simulink model "ev_ex_9"  (R2025a)
settings: Solver=VariableStepAuto  StartTime=0.0  StopTime=3600  RelTol=1e-3
undefined symbols (not defined in the file or in its folder): Ion, Lithium
libraries: spsBatteryLib x2, spsDiodeLib x2, spsIdealSwitchLib x2, spsSeriesRLCBranchLib x2, spsGroundLib x1, BatteryBalancing x1, sps_lib x1
settings Model: Creator=KRISHNA  LastModifiedBy=KRISHNA

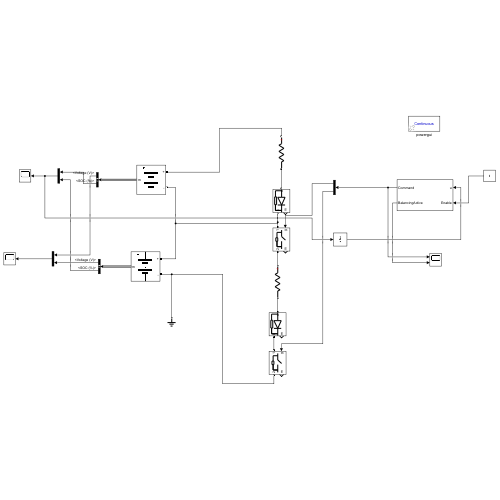
[thumbnail: Simulink's stored preview of the top-level diagram]
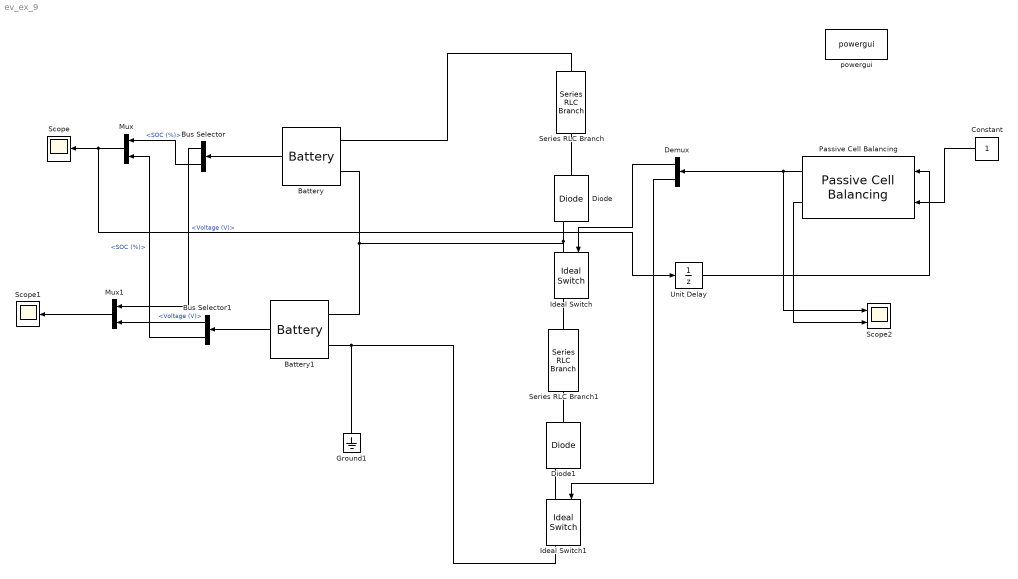
== system ev_ex_9 ==
  Battery : spsBatteryLib/Battery  BatType=Lithium-Ion  NomV=7.2  NomQ=5.4  SOC=90  Batt_Tr=1  PresetModel=on  MaxQ=5.4  MinV=5.4  FullV=8.3807  Dis_rate=2.3478  R=0.013333  Normal_OP=4.8835  expZone="[7.7788      0.2653]"
  Battery1 : spsBatteryLib/Battery  BatType=Lithium-Ion  NomV=7.2  NomQ=5.4  SOC=70  Batt_Tr=1  PresetModel=on  MaxQ=5.4  MinV=5.4  FullV=8.3807  Dis_rate=2.3478  R=0.013333  Normal_OP=4.8835  expZone="[7.7788      0.2653]"
  Bus Selector : BusSelector  OutputSignals=Voltage (V),SOC (%)
  Bus Selector1 : BusSelector  OutputSignals=Voltage (V),SOC (%)
  Constant : Constant
  Demux : Demux  Outputs=2
  Diode : spsDiodeLib/Diode  Ron=0.001  Lon=0  Vf=0.8  IC=0  UseSnubber=0  Rs=500  Cs=250e-9  Measurements=on
  Diode1 : spsDiodeLib/Diode  Ron=0.001  Lon=0  Vf=0.8  IC=0  UseSnubber=0  Rs=500  Cs=250e-9  Measurements=on
  Ground1 : spsGroundLib/Ground  LConnTagsString=a
  Ideal Switch : spsIdealSwitchLib/Ideal Switch  Ron=0.001  Lon=0  IC=0  Rs=1e5  Cs=inf  Measurements=on
  Ideal Switch1 : spsIdealSwitchLib/Ideal Switch  Ron=0.001  Lon=0  IC=0  Rs=1e5  Cs=inf  Measurements=on
  Mux : Mux  Inputs=2
  Mux1 : Mux  Inputs=2
  Passive Cell Balancing : BatteryBalancing/Passive Cell Balancing  Threshold=0.2  HysteresisBand=0  Td_on=1  Td_off=1  Ts=1  dataType=double
      settings: LibrarySourceBlock=batt_sl_lib/Cell Balancing/Passive Cell Balancing
  Scope : Scope
      settings: ActiveDisplayYMinimum=-10.40273292213508  ActiveDisplayYMaximum=101.52121489807514
  Scope1 : Scope
      settings: ActiveDisplayYMinimum=-0.97308129227086171  ActiveDisplayYMaximum=8.7577316304377568
  Scope2 : Scope  NumInputPorts=2
      settings: ActiveDisplayYMinimum=-0.12499999999999997  ActiveDisplayYMaximum=1.125  DataLoggingVariableName=ScopeData2
  Series RLC Branch : spsSeriesRLCBranchLib/Series RLC Branch  LConnTagsString=__new0  RConnTagsString=__new0  BranchType=R  Resistance=1  Inductance=1e-3  SetiL0=off  InitialCurrent=0  Capacitance=1e-6  Setx0=off  InitialVoltage=0  Measurements=None
  Series RLC Branch1 : spsSeriesRLCBranchLib/Series RLC Branch  LConnTagsString=__new0  RConnTagsString=__new0  BranchType=R  Resistance=1  Inductance=1e-3  SetiL0=off  InitialCurrent=0  Capacitance=1e-6  Setx0=off  InitialVoltage=0  Measurements=None
  Unit Delay : UnitDelay  SampleTime=-1  HasFrameUpgradeWarning=on
  powergui : sps_lib/powergui  Priority=1  SimulationMode=Continuous  SampleTime=50e-6  frequency=60  Iterations=50  frequencyindice=0  Pbase=100e6  ErrMax=1e-4  UnitsV=kV  UnitsW=MW  buscounter=0  FunctionMessages=off  echomessages=off  EnableUseOfTLC=off  CurrentSourceSwitches=off  DisableSnubberDevices=off  DisableRonSwitches=off  DisableVfSwitches=off  DisplayEquations=off  AutomaticDiscreteSolvers=off  SolverType=Tustin/Backward Euler (TBE)  Interpol=off  ExternalGateDelay=off  methode=off  Ts=100  x0status=blocks  SPID=on  SwTol=0  HookPort=off  NonlinearTolerance=1e-4  nMaxIteration=100  ContinueOnMaxIteration=off  RestoreLinks=warning  ResistiveCurrentMeasurement=off  Frange=[0:2:500]  Ylog=off  Xlog=on  ShowGrid=off  save=off  variable=ZData  structure=0  ZoomFFT=off  StartTime=0.0  cycles=1  DisplayStyle=1  fundamental=60  FreqAxis=off  MaxFrequency=1000  frequencyindicesteady=1  RmsSteady=1  display=off
  wires:
  Constant/1 -> Passive Cell Balancing/2
  Mux1/1 -> Scope1/1
  Mux/1 -> Unit Delay/1, Scope/1
  Bus Selector/2 -> Mux/1  "<SOC (%)>"
  Bus Selector/1 -> Mux1/1  "<Voltage (V)>"
  Battery1/1 -> Bus Selector1/1
  Bus Selector1/2 -> Mux/2  "<SOC (%)>"
  Bus Selector1/1 -> Mux1/2  "<Voltage (V)>"
  Battery/1 -> Bus Selector/1
  Demux/1 -> Ideal Switch/1
  Demux/2 -> Ideal Switch1/1
  Passive Cell Balancing/1 -> Scope2/1, Demux/1
  Passive Cell Balancing/2 -> Scope2/2
  Unit Delay/1 -> Passive Cell Balancing/1
  connections:
  Series RLC Branch/LConn1 -- Battery/LConn1
  Diode/LConn1 -- Series RLC Branch/RConn1
  Battery1/LConn1 -- Battery/LConn2 -- Diode/RConn1 -- Ideal Switch/LConn1
  Series RLC Branch1/LConn1 -- Ideal Switch/RConn1
  Diode1/LConn1 -- Series RLC Branch1/RConn1
  Ideal Switch1/LConn1 -- Diode1/RConn1
  Ideal Switch1/RConn1 -- Ground1/LConn1 -- Battery1/LConn2
